simulink model "LQG_test"  (R2015a)
settings: Solver=ode5  StartTime=0.0  StopTime=14  FixedStep=1e-4  RelTol=1e-3
values from neighbouring files (symbols this model uses):
  A = [-2498.14110998 -1127.91157577 -580.133219002 831.739808787 -469.393375659 -335.144039613 1431.44660589 426.118931463 -192.073592472 863.339278026 250.29301897 -203.532501061 ... (36 elements, 6x6)]    [Identified.mat]    (also in Identified2.mat = [-1.86629128978 -487.895153008 0 0 0 0 487.854565442 -1.8892; Identified3_real_inputs.mat = [125.649383136 -1075.44985766 0 0 0 0 236.024000906 -128.804; main_matlab.m = A(1:4,1:4))
  B = [234.044446428 182.655871798 229.451997242 -257.769990537 6.41427392218 -2.36072977801 -56.7379037546 -6.1159558257 103.458552161 -98.9688585342 -31.472523392 -27.7002611695 ... (18 elements, 6x3)]    [Identified.mat]    (also in Identified2.mat = [4.85156912923 0.611386220144 13.2516502255 7.37441612073 0.; Identified3_real_inputs.mat = [-913.807005742 -1063.47882704 226.197070552 -293.138793165 ; main_matlab.m = B(1:4,:))
  C = [0.558614590312  -0.34058227307  0.150866976372  -0.526807567749  1.58511664422  0.919119471275; -0.877431644416  0.31517377346  1.7154523531  1.21632251562  -4.09823482119  -1.94089288318]    [Identified.mat]    (also in Identified2.mat = [0.0985270561708  -0.284150162317  1.93097917616  -0.0121498; Identified3_real_inputs.mat = [-0.0510975239854  0.0401880943917  -0.0900037144493  -0.119; main_matlab.m = C(:,1:4))
  H = H(1:4,:)    [main_matlab.m]
libraries: simulink x1, cstblocks x1
settings Model: Creator=p4wp4w  LastModifiedBy=p4wp4w

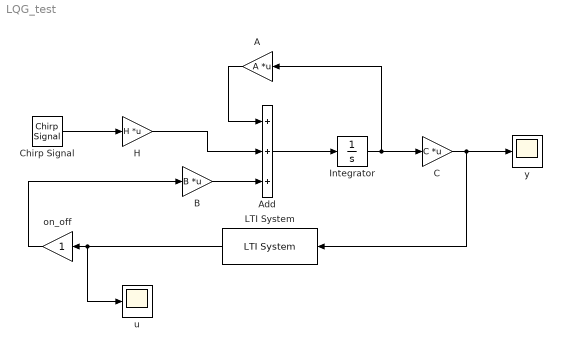
== system LQG_test ==
  A : Gain  Gain=A  Multiplication=Matrix(K*u)
  Add : Sum  Inputs=+++
  B : Gain  Gain=B  Multiplication=Matrix(K*u)
  C : Gain  Gain=C  Multiplication=Matrix(K*u)
  Chirp Signal : simulink/Sources/Chirp Signal  f1=0.1  T=14  f2=140
  H : Gain  Gain=H  Multiplication=Matrix(K*u)
  Integrator : Integrator
  LTI System : cstblocks/LTI System  sys=rlqg  IC=[]
  on_off : Gain
  u : Scope
  y : Scope
  wires:
  Add/1 -> Integrator/1
  A/1 -> Add/1
  B/1 -> Add/3
  Integrator/1 -> C/1, A/1
  C/1 -> y/1, LTI System/1
  H/1 -> Add/2
  Chirp Signal/1 -> H/1
  on_off/1 -> B/1
  LTI System/1 -> u/1, on_off/1
